simulink model "neuron1"  (R2015a)
settings: Solver=ode4  StartTime=0.0  StopTime=200  FixedStep=0.01  RelTol=1e-3
values from neighbouring files (symbols this model uses):
  J1 = Jr + mw * r*r    (= 0.541666666667)    [LP1.m]    (also in ParametryDoSymulacji.m = 0.416666666667; USImodel.m = 0.416666666667; wskaJak1.m = 0.416666666667; wskaJak2.m = 0.416666666667)
  J2 = Jr + mw * r*r    (= 0.541666666667)    [ParametryDoSymulacji.m]    (also in USImodel.m; wskaJak1.m; wskaJak2.m; wskaJak3.m)
  k = 0.1    [LP1.m]    (also in ParametryDoSymulacji.m; USImodel.m; wskaJak1.m; wskaJak2.m)
  ke = 5    [LP1.m]    (also in ParametryDoSymulacji.m; USImodel.m; wskaJak1.m; wskaJak2.m)
  L = 0.1    [LP1.m]    (also in ParametryDoSymulacji.m; USImodel.m; wskaJak1.m; wskaJak2.m)
  R = 2    [LP1.m]    (also in ParametryDoSymulacji.m; USImodel.m; wskaJak1.m; wskaJak2.m)
undefined symbols (not defined in the file or in its folder): sigbuilder_block, W
settings Model: Creator=Student  LastModifiedBy=konra

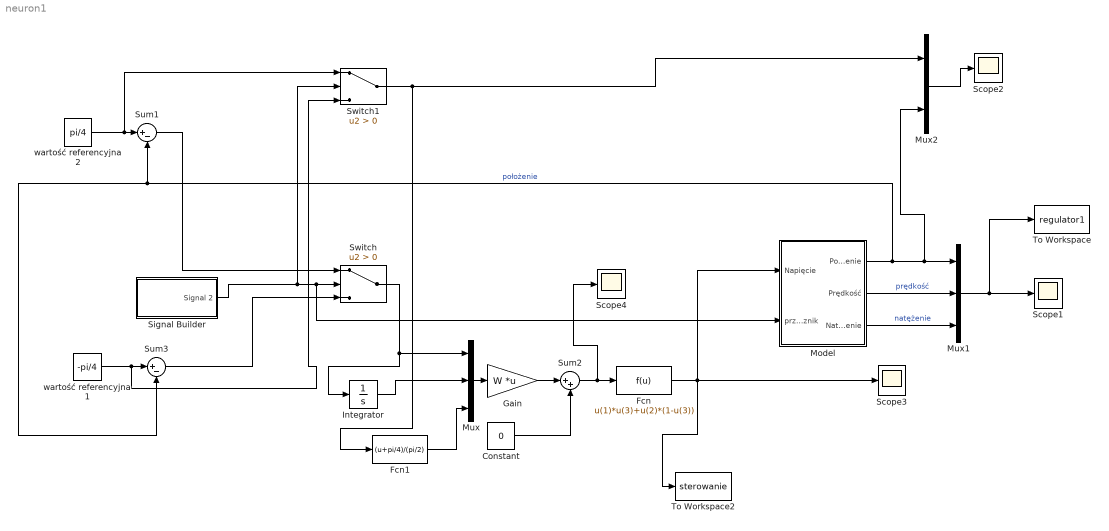
== system neuron1 ==
  Constant : Constant  Value=0
  Fcn : Fcn  Expr=u(1)*u(3)+u(2)*(1-u(3))
  Fcn1 : Fcn  Expr=(u+pi/4)/(pi/2)
  Gain : Gain  Gain=W  Multiplication=Matrix(K*u) (u vector)
  Integrator : Integrator
  Model : Subsystem
  Mux : Mux  Inputs=3
  Mux1 : Mux  Inputs=3
  Mux2 : Mux  Inputs=2
  Scope{1..4} (4 alike) : Scope
      Scope1 settings: ShowLegends=on  MaxDataPoints=10000
      Scope2 settings: ShowLegends=on  MaxDataPoints=10000
      Scope3 settings: SaveName=ScopeData3
      Scope4 settings: SaveName=ScopeData2
  Signal Builder : Subsystem  Tag=STV Subsys  LoadFcn=sigbuilder_block('load');  StartFcn=sigbuilder_block('start');  StopFcn=sigbuilder_block('stop');  ClipboardFcn=sigbuilder_block('clipboard');  mask(Sigbuilder block){}
      mask help: Simulink:masks:SigbuilderBlock_MD
      mask init:
      | if ~strcmp(get_param(bdroot(gcbh),'SimulationStatus'),'stopped') tuvar = sigbuilder_block('maskInit'); end
      settings: CopyFcn=sigbuilder_block('copy');  DeleteFcn=sigbuilder_block('delete');  ModelCloseFcn=sigbuilder_block('modelClose');  PreSaveFcn=sigbuilder_block('preSave');  PauseFcn=sigbuilder_block('pause');  ContinueFcn=sigbuilder_block('continue');  NameChangeFcn=sigbuilder_block('namechange');  OpenFcn=sigbuilder_block('open',[437.6 199.2 550.4 400 ]);  CloseFcn=sigbuilder_block('close');
      mask Display: plot(0, 0, 100, 100,[2, 2, 32, 32, 2], [68, 8, 8, 68, 68],[32, 2], [38, 38], [32, 19, 2],[53, 60, 44], [32, 17, 17, 2],[16, 16, 31, 31]);txt = getActiveGroup(gcbh);text(2, 100, txt,'verticalAlignment', 'top');
  Sum1 : Sum  Inputs=|+-
  Sum2 : Sum  Inputs=|++
  Sum3 : Sum  Inputs=|+-
  Switch : Switch  Criteria=u2 > Threshold
  Switch1 : Switch  Criteria=u2 > Threshold
  To Workspace : ToWorkspace  VariableName=regulator1  SaveFormat=Structure With Time  SampleTime=-1
  To Workspace2 : ToWorkspace  VariableName=sterowanie  SaveFormat=Structure With Time  SampleTime=-1
  wartość referencyjna 1 : Constant  Value=-pi/4
  wartość referencyjna 2 : Constant  Value=pi/4
  wires:
  wartość referencyjna 2/1 -> Switch1/1, Sum1/1
  Model/3("Natężenie ") -> Mux1/3  "natężenie"
  Model/2(Prędkość) -> Mux1/2  "prędkość"
  Mux1/1 -> To Workspace/1, Scope1/1
  Sum1/1 -> Switch/1
  Mux/1 -> Gain/1
  Gain/1 -> Sum2/1
  Constant/1 -> Sum2/2
  Sum2/1 -> Scope4/1, Fcn/1
  Fcn/1 -> Model/1(Napięcie), Scope3/1, To Workspace2/1
  Integrator/1 -> Mux/2
  wartość referencyjna 1/1 -> Switch1/3, Sum3/1
  Model/1(Położenie) -> Sum3/2, Sum1/2, Mux2/2, Mux1/1  "położenie"
  Sum3/1 -> Switch/3
  Switch/1 -> Integrator/1, Mux/1
  Signal Builder/1(Signal 2) -> Switch1/2, Model/2(przelacznik), Switch/2
  Mux2/1 -> Scope2/1
  Switch1/1 -> Fcn1/1, Mux2/1
  Fcn1/1 -> Mux/3

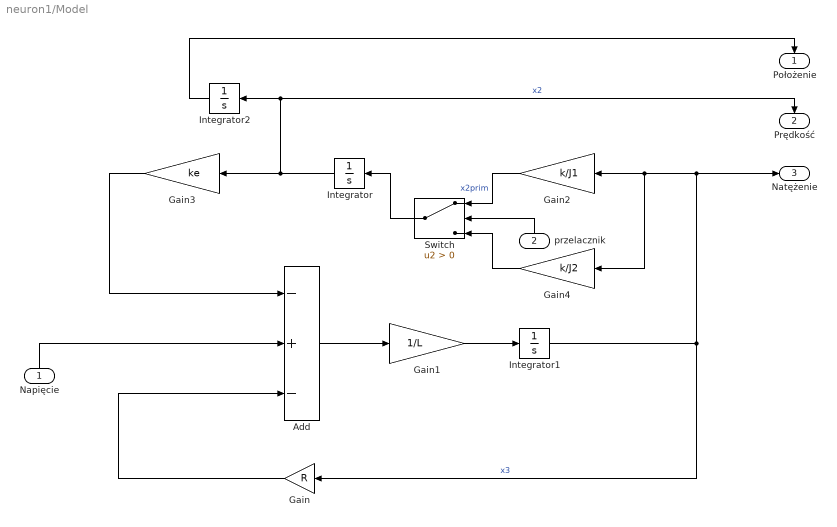
== system neuron1/Model ==
  Napięcie : Inport
  przelacznik : Inport  Port=2
  Add : Sum  Inputs=-+-
  Gain : Gain  Gain=R
  Gain1 : Gain  Gain=1/L
  Gain2 : Gain  Gain=k/J1
  Gain3 : Gain  Gain=ke
  Gain4 : Gain  Gain=k/J2
  Integrator : Integrator
  Integrator1 : Integrator
  Integrator2 : Integrator  InitialCondition=-pi/4
  Switch : Switch  Criteria=u2 > Threshold
  Położenie : Outport
  Prędkość : Outport  Port=2
  "Natężenie " : Outport  Port=3
  wires:
  Add/1 -> Gain1/1
  Gain1/1 -> Integrator1/1
  Gain3/1 -> Add/1
  Integrator/1 -> Prędkość/1, Integrator2/1, Gain3/1  "x2"
  Integrator2/1 -> Położenie/1
  Gain/1 -> Add/3
  Integrator1/1 -> "Natężenie "/1, Gain4/1, Gain2/1, Gain/1  "x3"
  Napięcie/1 -> Add/2
  Gain4/1 -> Switch/3
  Gain2/1 -> Switch/1  "x2prim"
  Switch/1 -> Integrator/1
  przelacznik/1 -> Switch/2

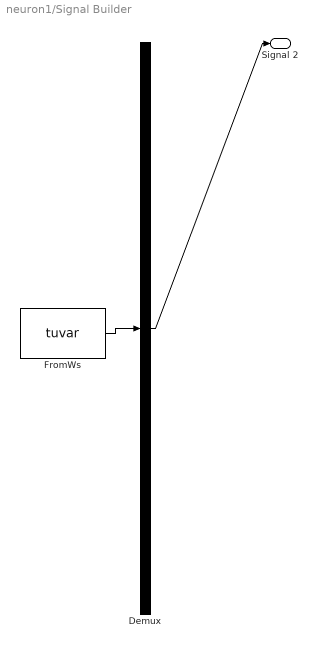
== system neuron1/Signal Builder ==
  Demux : Demux  Tag=STV Demux  Outputs=1
  FromWs : FromWorkspace  Tag=STV FromWs  VariableName=tuvar  SampleTime=0
      SigBuilderData=|
      | common.afterFinalStr = 'Extrapolate'
      | common.sampleTime = 0
      | dataSet.timeRange = [0 200]
      | dataSet.name = 'Group 1'
      | sbobj.Groups.Name = 'Group 1'
      | sbobj.Groups.Signals.Name = 'Signal 2'
      | sbobj.Groups.Signals.XData = [0 50 50 100 100 150 150 200]
      | sbobj.Groups.Signals.YData = [1 1 0 0 1 1 0 0]
      | sbobj.Groups.TimeRange = [0 200]
  Signal 2 : Outport  Tag=STV Outport
  wires:
  FromWs/1 -> Demux/1
  Demux/1 -> Signal 2/1
